simulink model "step2"  (R2021a)
settings: Solver=VariableStepAuto  StartTime=0.0  StopTime=10.0  RelTol=1e-3
settings Model: Creator=konsta  LastModifiedBy=konsta

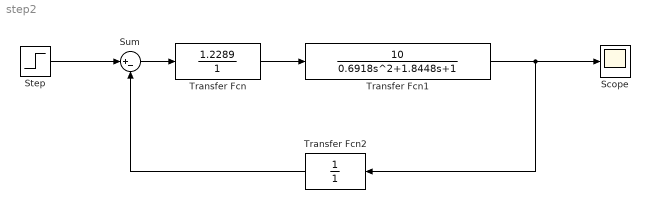
== system step2 ==
  Scope : Scope
  Step : Step  After=10  SampleTime=0
  Sum : Sum  Inputs=|+-
  Transfer Fcn : TransferFcn  Numerator=[1.2289]  Denominator=[0 1]
  Transfer Fcn1 : TransferFcn  Numerator=[10]  Denominator=[0.6918 1.8448 1]
  Transfer Fcn2 : TransferFcn  Denominator=[0 1]
  wires:
  Transfer Fcn/1 -> Transfer Fcn1/1
  Transfer Fcn1/1 -> Transfer Fcn2/1, Scope/1
  Sum/1 -> Transfer Fcn/1
  Step/1 -> Sum/1
  Transfer Fcn2/1 -> Sum/2
